simulink model "MotorTorqueControlTest_working_5_8_2022_ADC_FILT_Mo"  (R2024b)
settings: Solver=FixedStepAuto  StartTime=0.0  StopTime=inf  FixedStep=0.001  RelTol=1e-3  EnableMultiTasking=on
undefined symbols (not defined in the file): mu_X, mu_y, sigma_X, sigma_y
libraries: slrealtimeethercatlib x35, slrealtimeiplib x6, slrealtimeutilitieslib x5, simulink_extras x5, slrealtimeloglib x3, slpidlib x1, simulink x1
(part 1 of 4)
settings Model: SimulationMode=external  ExtModeEnableFloating=off  Creator=mbout  LastModifiedBy=Andy
settings SolverCC: ConcurrentTasks=on  AlgebraicLoopSolver=TrustRegion  PositivePriorityOrder=on  AutoInsertRateTranBlk=on  InsertRTBMode=Never (minimum delay)
settings DataIOCC: SaveFormat=Array  SaveState=on  SignalLoggingName=logsOut
settings OptimizationCC: BlockReduction=off  BooleanDataType=off  OptimizeBlockIOStorage=off  BufferReuse=off  ReuseModelBlockBuffer=off  GlobalBufferReuse=off  ExpressionFolding=off  LocalBlockOutputs=off  InitFltsAndDblsToZero=on  OptimizeDataStoreBuffers=off  BusAssignmentInplaceUpdate=off
settings DebuggingCC: SaveWithParameterizedLinksMsg=none  UnderspecifiedInitializationDetection=Classic  MergeDetectMultiDrivingBlocksExec=none  CheckExecutionContextPreStartOutputMsg=on  SignalResolutionControl=TryResolveAllWithWarning  TasksWithSamePriorityMsg=none  ParameterPrecisionLossMsg=none  UnconnectedInputMsg=warning  UnconnectedOutputMsg=warning  UnconnectedLineMsg=warning  SFUnexpectedBacktrackingDiag=warning  SFNoUnconditionalDefaultTransitionDiag=warning  SFExecutionAtInitializationDiag=none  UnderSpecifiedDimensionMsg=warning  ArithmeticOperatorsInVariantConditions=warning
settings HardwareCC: ProdBitPerLong=64  ProdLongLongMode=on  ProdHWDeviceType=Intel->x86-64 (Linux 64)
settings ModelReferenceCC: EnableRefExpFcnMdlSchedulingChecks=on  PropagateSignalLabelsOutOfModel=off
settings SFSimCC: SimUseLocalCustomCode=off  SimTargetLang=C++
settings RTWCC: Description=Speedgoat Real-Time Target Machine  SystemTargetFile=speedgoat.tlc  TemplateMakefile=slrealtime_default_tmf  RTWUseLocalCustomCode=off  Toolchain=Simulink Real-Time Toolchain  BuildConfiguration=Faster Runs  CodeExecutionProfiling=on  TargetLang=C++  GPUComputeCapability=3.5  DLArmComputeVersion=19.05
settings CodeAppCC: StateflowObjectComments=on
settings SimulinkRealTimeTargetCC: InstructionSetFMA=off  LogToMDFFile=off  SLRTFileLogMaxRuns=20
settings ConfigComp: CovMetricSettings=dw  CovSaveCumulativeToWorkspaceVar=on  CovSaveSingleToWorkspaceVar=on  CovExternalEMLEnable=off  CovSFcnEnable=off

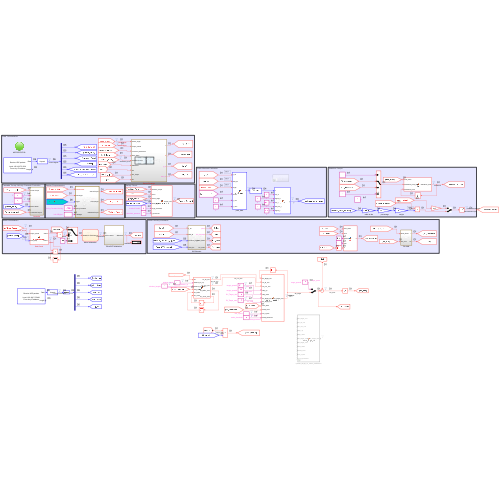
[thumbnail: Simulink's stored preview of the top-level diagram]
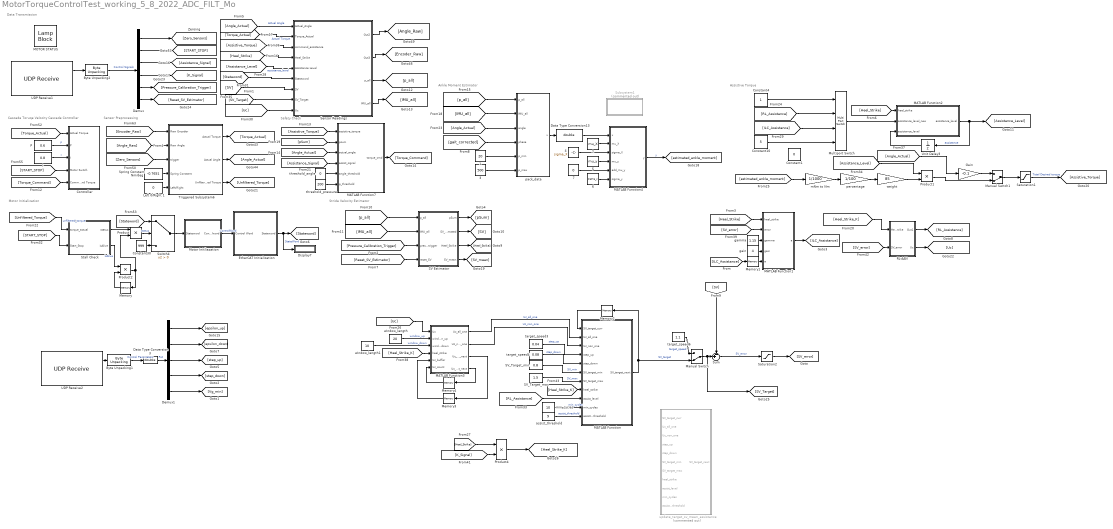
== system MotorTorqueControlTest_working_5_8_2022_ADC_FILT_Mo ==
  note: Ankle Moment Estimator
  note: Cascade Toruqe Velocity Cascade Controller
  note: Data Transmission
  note: Motor Initialization
  note: Sensor Preprocessing
  note: Stride Velocity Estimator
  note: Assistive Torque
  note: Safety Check
  1 : Constant  Value=20
  2 : Constant  Value=mu_X
  3 : Constant  Value=500
  4 : Constant  Value=sigma_X
  5 : Constant  Value=mu_y
  6 : Constant  Value=sigma_y
  7 : Constant  Value=0
  Byte Unpacking1 : slrealtimeutilitieslib/Byte Unpacking  MaskUnpackedDataTypes={['single']}  MaskUnpackedDataSizes={[6]}  MaskAlignment=1
  Byte Unpacking2 : slrealtimeutilitieslib/Byte Unpacking  MaskUnpackedDataTypes={['single']}  MaskUnpackedDataSizes={[6]}  MaskAlignment=1
  Constant1 : Constant  Value=0
  Constant10 : Constant  Value=5
  Constant30 : Constant  Value=999
  Constant4 : Constant
  Controller : Subsystem
  Data Type Conversion13 : DataTypeConversion  OutDataTypeStr=double  SaturateOnIntegerOverflow=off  RndMeth=Floor
  Data Type Conversion3 : DataTypeConversion  OutDataTypeStr=double  SaturateOnIntegerOverflow=off  RndMeth=Floor
  Demux : Demux  Outputs=6
  Demux1 : Demux  Outputs=5
  Display7 : Display
  EtherCAT Initialization : Subsystem
  Gain : Gain  Gain=-0.1
  I : Constant  Value=0.8
  Left 0/Right 1 : Constant  Value=0
  MATLAB Function : MATLAB Function  TreatAsAtomicUnit=on
  MATLAB Function1 : MATLAB Function  TreatAsAtomicUnit=on
  MATLAB Function2 : MATLAB Function  TreatAsAtomicUnit=on
  MATLAB Function3 : MATLAB Function  TreatAsAtomicUnit=on
  MATLAB Function4 : MATLAB Function  TreatAsAtomicUnit=on  SystemSampleTime=0.01
  MATLAB Function7 : MATLAB Function  TreatAsAtomicUnit=on  SystemSampleTime=0.001
  MOTOR STATUS : LampBlock  LabelPosition=Hide
  Manual Switch : ManualSwitch  CurrentSetting=0
  Manual Switch1 : ManualSwitch  CurrentSetting=0
  Memory : Memory  InitialCondition=1
  Memory1 : Memory
  Memory2 : Memory  InitialCondition=0.5
  Memory3 : Memory  InitialCondition=zeros(60,1)
  Memory4 : Memory  InitialCondition=zeros(2,1)
  Motor Initliazation : Stateflow chart  TreatAsAtomicUnit=on
  Multiport Switch : MultiPortSwitch  SaturateOnIntegerOverflow=off  InputSameDT=off
  P : Constant  Value=0.6
  Product{,1..2,4} (4 alike) : Product
  RL-AAN : Subsystem
  SV Estimator : Subsystem
  SV_Target_max : Constant  Value=1.5
  SV_Target_min : Constant  Value=0.8
  Saturation1 : Saturate  UpperLimit=8  LowerLimit=0
  Saturation2 : Saturate  UpperLimit=inf  LowerLimit=0
  Sensor Readings : Subsystem
  Spring Constant Nm/deg : Constant  Value=-0.7651
  Stall Check : MATLAB Function  TreatAsAtomicUnit=on
  Subsystem1 : Subsystem  Commented=on
  Sum : Sum  Inputs=-+|
  Switch4 : Switch  Criteria=u2 > Threshold  SaturateOnIntegerOverflow=off  InputSameDT=off
  Triggered Subsystem6 : Subsystem  TreatAsAtomicUnit=on
  UDP Receive1 : slrealtimeiplib/UDP Receive  useHostTargetConn=off  ipAddress=192.168.7.5  localPort=5431  rcvWidth=24  rcvFmAny=on  fmAddress='10.10.10.10'  sampleTime=0.1  enableMessage=off  maxPackets=1
  UDP Receive2 : slrealtimeiplib/UDP Receive  useHostTargetConn=off  ipAddress=192.168.7.5  localPort=5430  rcvWidth=24  rcvFmAny=on  fmAddress='10.10.10.10'  sampleTime=0.1  enableMessage=off  maxPackets=1
  Unit Delay3 : UnitDelay  SampleTime=-1
  assist_threshold : Constant  Value=9
  gain : Constant  Value=4
  gamma : Constant  Value=1.15
  mNm to Nm : Gain  Gain=1/1000
  min_cycles : Constant  Value=10
  pack_data : MATLAB Function  TreatAsAtomicUnit=on  SystemSampleTime=0.01
  percentage : Gain  Gain=1/100
  target_speed3 : Constant  Value=0.04
  target_speed4 : Constant  Value=0.08
  target_speed6 : Constant  Value=1.1
  threshold_angle : Constant  Value=0
  threshold_pressure : Constant  Value=200
  update_target_sv_mean_assistance : MATLAB Function  Commented=on  TreatAsAtomicUnit=on
  weight : Gain  Gain=85
  window_length : Constant  Value=20
  window_length1 : Constant  Value=10
  wires:
  EtherCAT Initialization/1(Stateword) -> [Stateword], Display7/1  "StateWord"
  [Zero_Sensors] -> Triggered Subsystem6/3(trigger)
  Sensor Readings/2(Out3) -> [Encoder_Raw]
  Triggered Subsystem6/2(Actual Angle) -> [Angle_Actual]
  Motor Initliazation/1(Controlword) -> EtherCAT Initialization/1(Control Word)  "ControlWord"
  [Encoder_Raw] -> Triggered Subsystem6/1(Raw Encoder)
  [Torque_Actual] -> Controller/1(Actual Torque)
  [START_STOP] -> Controller/4(Motor Switch)
  [Angle_Raw] -> Triggered Subsystem6/2(Raw Angle)
  Sensor Readings/1(Out2) -> [Angle_Raw]
  [Stateword] -> Switch4/1
  Constant30/1 -> Switch4/3
  P/1 -> Controller/2(P)  "P"
  I/1 -> Controller/3(I)  "I"
  MATLAB Function7/1(torque_cmd) -> [Torque_Command]
  Triggered Subsystem6/1(Actual Torque) -> [Torque_Actual]
  Saturation1/1 -> [Assistive_Torque]  "Total Desired torque"
  gain/1 -> MATLAB Function1/4(gain)
  gamma/1 -> MATLAB Function1/3(gamma)
  [SV] -> Sum/1
  Memory1/1 -> MATLAB Function1/5("a ")
  MATLAB Function1/1(a) -> [ILC_Assistance]
  [Angle_Actual] -> Sensor Readings/1(Actual_Angle)  "Actual Angle"
  [Torque_Actual] -> Sensor Readings/2(Torque_Actual)  "Actual Torque"
  percentage/1 -> weight/1
  [Assistive_Torque] -> Sensor Readings/3(command_assistance)
  mNm to Nm/1 -> percentage/1
  weight/1 -> Product1/2
  [RL_Assistance] -> Multiport Switch/2
  MATLAB Function4/1(y) -> [estimated_ankle_moment]  "y"
  Sensor Readings/3(p_all) -> [p_all]
  Sensor Readings/4(IMU_all) -> [IMU_all]
  [p_all] -> pack_data/1(p_all)
  [Angle_Actual] -> pack_data/3(angle)
  [gait_corrected] -> pack_data/4(phase)
  1/1 -> pack_data/5(p_min)
  3/1 -> pack_data/6(p_max)
  [estimated_ankle_moment] -> mNm to Nm/1
  MATLAB Function2/1(assistance_level) -> [Assistance_Level], Unit Delay3/1  "assistance"
  Unit Delay3/1 -> MATLAB Function2/3("assistance_level ")
  [Assistance_Level] -> Sensor Readings/5(Assistance Level)  "assistance_level"
  Constant10/1 -> Multiport Switch/4
  2/1 -> MATLAB Function4/2(mu_X)
  4/1 -> MATLAB Function4/3(sigma_X)
  5/1 -> MATLAB Function4/4(mu_y)
  6/1 -> MATLAB Function4/6(sigma_y)
  7/1 -> MATLAB Function4/5(add_mu_y)
  pack_data/1(x) -> Data Type Conversion13/1
  Data Type Conversion13/1 -> MATLAB Function4/1(x)
  [ILC_Assistance] -> Multiport Switch/3
  [Heel_Strike] -> MATLAB Function1/1(heel_strike)
  [IMU_all] -> pack_data/2(IMU_all)
  [START_STOP] -> Stall Check/2(Start_Stop)
  [Unfiltered_Torque] -> Stall Check/1(torque_actual)  "unfiltered_torque"
  Byte Unpacking2/1 -> Demux/1  "Control Signals"
  Demux/1 -> [Zero_Sensors]
  Demux/2 -> [START_STOP]
  Demux/3 -> [Assistance_Signal]
  Demux/4 -> [K_Signal]
  [Stateword] -> Sensor Readings/6(Stateword)
  UDP Receive1/1 -> Byte Unpacking2/1
  Demux/6 -> [Reset_SV_Estimator]
  Demux/5 -> [Pressure_Calibration_Trigger]
  [Heel_Strike] -> Sensor Readings/4(Heel_Strike)
  [Assistance_Level] -> Product1/1
  Constant4/1 -> Multiport Switch/1
  Multiport Switch/1 -> MATLAB Function2/2(assistance_level_new)
  [Heel_Strike] -> MATLAB Function2/1(heel_strike)
  [SV_error] -> MATLAB Function1/2(error)
  Saturation2/1 -> [SV_error]
  Sum/1 -> Saturation2/1  "SV_error"
  SV_Target_max/1 -> MATLAB Function/7(SV_target_max)  "SV_max"
  [SV_error] -> RL-AAN/2(SV_error)
  RL-AAN/1(Out1) -> [RL_Assistance]
  [Pressure_Calibration_Trigger] -> SV Estimator/3(pressure_trigger)
  [Reset_SV_Estimator] -> SV Estimator/4(reset_SV)
  SV Estimator/1(pSum) -> [pSum]
  SV Estimator/3(Heel_Strike) -> [Heel_Strike]
  SV Estimator/2(SV_estimated) -> [SV]
  [p_all] -> SV Estimator/1(p_all)
  [IMU_all] -> SV Estimator/2(IMU_all)
  [Torque_Command] -> Controller/5(Command Torque)
  Spring Constant Nm/deg/1 -> Triggered Subsystem6/4(Spring Constant)
  Switch4/1 -> Motor Initliazation/1(Stateword)
  Stall Check/1(status) -> Product/1
  [pSum] -> MATLAB Function7/2(psum)
  [Angle_Actual] -> MATLAB Function7/3(actual_angle)
  [Assistance_Signal] -> MATLAB Function7/4(assist_signal)
  threshold_pressure/1 -> MATLAB Function7/6(p_threshold)
  threshold_angle/1 -> MATLAB Function7/5(angle_threshold)
  [Assistive_Torque] -> MATLAB Function7/1(assistive_torque)
  [ILC_Assistance] -> Memory1/1
  Left 0/Right 1/1 -> Triggered Subsystem6/5(Left/Right)
  MATLAB Function/1(SV_target_next) -> Manual Switch/2, Memory2/1  "SV_target"
  target_speed3/1 -> MATLAB Function/4(step_up)  "step_up"
  target_speed4/1 -> MATLAB Function/5(step_down)  "step_down"
  SV_Target_min/1 -> MATLAB Function/6(SV_target_min)  "SV_min"
  Demux1/2 -> [epsilon_down]
  Demux1/3 -> [step_up]
  Demux1/1 -> [epsilon_up]
  Demux1/4 -> [step_down]
  UDP Receive2/1 -> Byte Unpacking1/1
  Byte Unpacking1/1 -> Data Type Conversion3/1  "Control Parameters"
  Demux1/5 -> [Vg_min]
  Data Type Conversion3/1 -> Demux1/1  "Pot"
  [SV] -> Sensor Readings/7(SV)
  SV Estimator/4(SV_mean) -> [SV_mean]
  target_speed6/1 -> Manual Switch/1  "target_speed"
  Manual Switch/1 -> [SV_Target], Sum/2
  Triggered Subsystem6/3(Unfiltered Torque) -> [Unfiltered_Torque]
  Stall Check/2(isAlive) -> Product2/1  "isAlive"
  Memory/1 -> Product2/2
  Product2/1 -> Memory/1, Product/2
  Product/1 -> Switch4/2  "status"
  RL-AAN/2(Uc) -> [Uc]
  [Uc] -> MATLAB Function3/1(Uc)
  MATLAB Function3/3(Uc_buffer_next) -> Memory3/1
  Memory3/1 -> MATLAB Function3/5(Uc_buffer)
  window_length/1 -> MATLAB Function3/2(window_len_up)  "window_up"
  MATLAB Function3/2(Uc_non_one) -> MATLAB Function/3(Uc_non_one)  "Uc_non_one"
  MATLAB Function3/1(Uc_all_one) -> MATLAB Function/2(Uc_all_one)  "Uc_all_one"
  Memory2/1 -> MATLAB Function/1(SV_target_curr)
  MATLAB Function3/4(Uc_count_next) -> Memory4/1
  Memory4/1 -> MATLAB Function3/6(Uc_count)
  window_length1/1 -> MATLAB Function3/3(window_len_down)  "window_down"
  [SV_Target] -> Sensor Readings/8(SV_Target)
  [Uc] -> Sensor Readings/9(Uc)
  [K_Signal] -> Product4/2
  Product4/1 -> [Heel_Strike_K]
  [Heel_Strike] -> Product4/1
  [Heel_Strike_K] -> MATLAB Function3/4(heel_strike)
  [Heel_Strike_K] -> MATLAB Function/8(heel_strike)
  [Heel_Strike_K] -> RL-AAN/1(Heel_Strike)
  Product1/1 -> Manual Switch1/2
  min_cycles/1 -> MATLAB Function/10(min_cycles)  "min_cycles"
  assist_threshold/1 -> MATLAB Function/11(assist_threshold)  "assist_threshold"
  [RL_Assistance] -> MATLAB Function/9(assist_level)
  Manual Switch1/1 -> Saturation1/1
  Gain/1 -> Manual Switch1/1
  [Angle_Actual] -> Gain/1

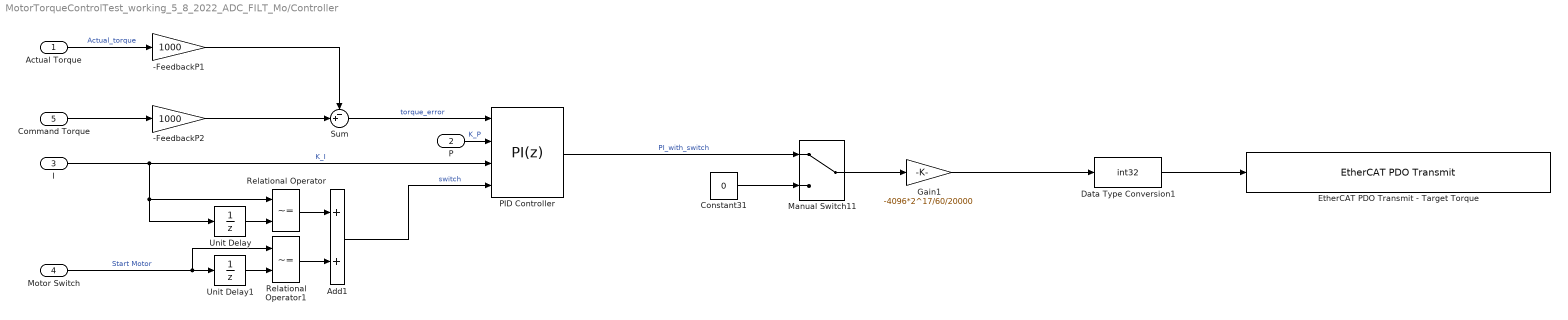
== system MotorTorqueControlTest_working_5_8_2022_ADC_FILT_Mo/Controller ==
  Actual Torque : Inport
  P : Inport  Port=2
  I : Inport  Port=3
  Motor Switch : Inport  Port=4
  Command Torque : Inport  Port=5
  -FeedbackP1 : Gain  Gain=1000
  -FeedbackP2 : Gain  Gain=1000
  Add1 : Sum
  Constant31 : Constant  Value=0
  Data Type Conversion1 : DataTypeConversion  OutDataTypeStr=int32  SaturateOnIntegerOverflow=off  RndMeth=Floor
  EtherCAT PDO Transmit - Target Torque : slrealtimeethercatlib/EtherCAT PDO Transmit  Priority=3  sig_name=Drive 1 (AMC Servo Drive).Outputs.Target Velocity  sig_offset=328  sig_type=int32  type_size=32  sig_dim=1  device_id=0  sample_time=0.001000
  Gain1 : Gain  Gain=-4096*2^17/60/20000
  Manual Switch11 : ManualSwitch
  PID Controller : slpidlib/PID Controller  Controller=PI  Form=Parallel  TimeDomain=Discrete-time  UseExternalTs=off  SampleTime=-1  IntegratorMethod=Forward Euler  FilterMethod=Forward Euler  ControllerParametersSource=external  P=1  I=1  UseKiTs=off  D=0  UseExternalDerivativeSource=off  N=100  UseFilter=on  TunerSelectOption=Transfer Function Based (PID Tuner App)  InitialConditionSource=internal  InitialConditionForIntegrator=0  InitialConditionForFilter=0  DifferentiatorICPrevScaledInput=0  ExternalReset=either  TrackingMode=off  Kt=1  LimitOutput=off  SatLimitsSource=internal  UpperSaturationLimit=50  LowerSaturationLimit=-50  LinearizeAsGain=on  AntiWindupMode=none  Kb=1  LimitIntegrator=off  UpperIntegratorSaturationLimit=inf  LowerIntegratorSaturationLimit=-inf  POutMin=[]  POutMax=[]  IOutMin=[]  IOutMax=[]  DOutMin=[]  DOutMax=[]  NOutMin=[]  NOutMax=[]  SumOutMin=[]  SumOutMax=[]  SaturationOutMin=[]  SaturationOutMax=[]  PParamMin=[]  PParamMax=[]  IParamMin=[]  IParamMax=[]  DParamMin=[]  DParamMax=[]  NParamMin=[]  NParamMax=[]  KbParamMin=[]  KbParamMax=[]  KtParamMin=[]  KtParamMax=[]  KbOutMin=[]  KbOutMax=[]  KtOutMin=[]  KtOutMax=[]  IntegratorOutMin=[]  IntegratorOutMax=[]  FilterOutMin=[]  FilterOutMax=[]  SumI1OutMin=[]  SumI1OutMax=[]  SumI2OutMin=[]  SumI2OutMax=[]  SumI3OutMin=[]  SumI3OutMax=[]  SumI4OutMin=[]  SumI4OutMax=[]  SumDOutMin=[]  SumDOutMax=[]  DifferentiatorOutMin=[]  DifferentiatorOutMax=[]  FilterDiffOutCoefMin=[]  FilterDiffOutCoefMax=[]  ReciprocalOutMin=[]  ReciprocalOutMax=[]  SumDenOutMin=[]  SumDenOutMax=[]  SumNumOutMin=[]  SumNumOutMax=[]  DivideOutMin=[]  DivideOutMax=[]  UdiffTsProdOutMin=[]  UdiffTsProdOutMax=[]  NTsProdOutMin=[]  NTsProdOutMax=[]  UintegralTsProdOutMin=[]  UintegralTsProdOutMax=[]  UngainTsProdOutMin=[]  UngainTsProdOutMax=[]  ClampingZeroOutDataTypeStr=Inherit: Inherit via back propagation  ClampingZeroOutMin=[]  ClampingZeroOutMax=[]  FilterDenConstantOutDataTypeStr=Inherit: Inherit via back propagation  FilterDenConstantOutMin=[]  FilterDenConstantOutMax=[]  PCopyOutDataTypeStr=Inherit: Inherit via back propagation  PCopyOutMin=[]  PCopyOutMax=[]  NCopyOutDataTypeStr=Inherit: Inherit via back propagation  NCopyOutMin=[]  NCopyOutMax=[]  IntegratorContinuousStateAttributes=''  IntegratorStateMustResolveToSignalObject=off  IntegratorRTWStateStorageClass=Auto  FilterContinuousStateAttributes=''  FilterStateMustResolveToSignalObject=off  FilterRTWStateStorageClass=Auto  ParallelPVariant=ExternalParameters  IdealPVariant=Disabled  IVariant=ExternalParameters  DVariant=Disabled  IntegratorVariant=Discrete  SatVariant=Disabled  AWVariant=Passthrough  PCopyVariant=Disabled  TRVariant=Disabled  FdbkBlocksVariant=Forward  IdealPFdbkVariant=Disabled  SatFdbkVariant=Disabled  DerivativeFilterVariant=Disabled  NVariant=Disabled  NCopyVariant=Disabled_SignalSpec  FilterICVariant=Disabled  IntegratorICVariant=InternalICs  ExternalResetVariant=ExternalReset  TRSumVariant=Passthrough  SumFdbkVariant=Disabled  SumVariant=Sum_PI  TsampFilterVariant=InternalTs  TsampNgainVariant=Passthrough  TsampIntegralVariant=Disabled_SignalSpec  ExternalSaturationOutDataTypeStr=Inherit: Same as second input  DerivativeSourceVariant=Disabled  PreIntVariant=InternalPreInt
  Relational Operator : RelationalOperator  Operator=~=  OutDataTypeStr=boolean  RndMeth=Simplest  InputSameDT=off
  Relational Operator1 : RelationalOperator  Operator=~=  OutDataTypeStr=boolean  RndMeth=Simplest  InputSameDT=off
  Sum : Sum  Inputs=-+|
  Unit Delay : UnitDelay  SampleTime=-1  HasFrameUpgradeWarning=on
  Unit Delay1 : UnitDelay  SampleTime=-1  HasFrameUpgradeWarning=on
  wires:
  Data Type Conversion1/1 -> EtherCAT PDO Transmit - Target Torque/1
  Motor Switch/1 -> Unit Delay1/1, Relational Operator1/1  "Start Motor"
  Unit Delay/1 -> Relational Operator/2
  Unit Delay1/1 -> Relational Operator1/2
  Relational Operator/1 -> Add1/1
  Relational Operator1/1 -> Add1/2
  Command Torque/1 -> -FeedbackP2/1
  -FeedbackP2/1 -> Sum/2
  -FeedbackP1/1 -> Sum/1
  Actual Torque/1 -> -FeedbackP1/1  "Actual_torque"
  I/1 -> Unit Delay/1, Relational Operator/1, PID Controller/3  "K_I"
  Sum/1 -> PID Controller/1  "torque_error"
  P/1 -> PID Controller/2  "K_P"
  Add1/1 -> PID Controller/4  "switch"
  PID Controller/1 -> Manual Switch11/1  "PI_with_switch"
  Constant31/1 -> Manual Switch11/2
  Manual Switch11/1 -> Gain1/1
  Gain1/1 -> Data Type Conversion1/1

== system MotorTorqueControlTest_working_5_8_2022_ADC_FILT_Mo/EtherCAT Initialization ==
  note: This block is used for the initialization of the EtherCAT network. The block points the model to the folder location of the ENI file created in TwinCAT. Note that the ENI file must also be present in the simulink's model directory, and the name of the ENI file must be different from the simulink model.
  note: This block and associated scope is used to show the state of the EtherCAT State Machine. Clicking "Help" in the Get State block shows the status numbers and their corresponding states. The scope can be helpful for determing the state and troubleshooting if the drive is not enabling and the motor is not turning on.
  note: This block and associated scope is used to show the status word of the drive's state machine. Note that the drive's state machine is different from the EtherCAT State Machine described above. This scope is also helpful for troubleshooting. Note that the status word is given as a decimal number and must be converted to binary to decipher its meaning.
  note: The control word is the PDO that changes the state of the motor. Refer to the EPOS library for more information.
  Control Word : Inport
  Constant2 : Constant  Value=9
  Data Type Conversion : DataTypeConversion  OutDataTypeStr=uint16  SaturateOnIntegerOverflow=off  RndMeth=Floor
  Data Type Conversion1 : DataTypeConversion  OutDataTypeStr=uint16  SaturateOnIntegerOverflow=off  RndMeth=Floor
  Display : Display
      settings: Format=hex (Stored Integer)
  Display1 : Display
  Display2 : Display
  EtherCAT Get State : slrealtimeethercatlib/EtherCAT Get State  device_id=0  sample_time=0
  EtherCAT Init : slrealtimeethercatlib/EtherCAT Init  Priority=0  config_file=C:\Users\Andy\Desktop\AFO\PDO__AMC_Drive_32_Input.xml  device_id=0  portnum=1  initstate=2  dctuning=2  enaDebug=1  logFile='c:\dbglog.txt'  sample_time=0.001000  DCMode=0
  EtherCAT PDO Receive : slrealtimeethercatlib/EtherCAT PDO Receive  Priority=2  sig_name=Drive 1 (AMC Servo Drive).Inputs.Status Word  sig_offset=312  sig_type=uint16  type_size=16  sig_dim=1  device_id=0  sample_time=0.001000
  EtherCAT PDO Transmit : slrealtimeethercatlib/EtherCAT PDO Transmit  Priority=3  sig_name=Drive 1 (AMC Servo Drive).Outputs.Control Word  sig_offset=312  sig_type=uint16  type_size=16  sig_dim=1  device_id=0  sample_time=0.001000
  EtherCAT PDO Transmit1 : slrealtimeethercatlib/EtherCAT PDO Transmit  Priority=3  sig_name=Drive 1 (AMC Servo Drive).Outputs.Modes of Operation  sig_offset=360  sig_type=uint16  type_size=16  sig_dim=1  device_id=0  sample_time=0.001000
  Stateword : Outport
  wires:
  EtherCAT PDO Receive/1 -> Stateword/1, Display2/1
  EtherCAT Get State/1 -> Display1/1
  EtherCAT Init/1 -> Display/1
  Data Type Conversion/1 -> EtherCAT PDO Transmit/1
  Control Word/1 -> Data Type Conversion/1
  Constant2/1 -> Data Type Conversion1/1
  Data Type Conversion1/1 -> EtherCAT PDO Transmit1/1

== system MotorTorqueControlTest_working_5_8_2022_ADC_FILT_Mo/RL-AAN ==
  Heel_Strike : Inport
  SV_error : Inport  Port=2
  Byte Unpacking1 : slrealtimeutilitieslib/Byte Unpacking  MaskUnpackedDataTypes={['double']}  MaskUnpackedDataSizes={[2]}  MaskAlignment=1
  Demux1 : Demux  Outputs=2
  RT : RateTransition  Deterministic=off  OutPortSampleTime=0.001
  Saturation : Saturate  UpperLimit=10  LowerLimit=0
  Triggered Subsystem : Subsystem  TreatAsAtomicUnit=on
  UDP RL_AAN : slrealtimeiplib/UDP Receive  useHostTargetConn=off  ipAddress=192.168.7.5  localPort=6009  rcvWidth=16  rcvFmAny=on  fmAddress='10.10.10.10'  sampleTime=0.1  enableMessage=off  maxPackets=1
  Out1 : Outport
  Uc : Outport  Port=2
  wires:
  SV_error/1 -> Triggered Subsystem/1(In1)
  Heel_Strike/1 -> Triggered Subsystem/Trigger
  Saturation/1 -> Out1/1  "RL_AAN"
  Byte Unpacking1/1 -> RT/1
  UDP RL_AAN/1 -> Byte Unpacking1/1
  Demux1/1 -> Saturation/1
  Demux1/2 -> Uc/1  "Uc"
  RT/1 -> Demux1/1

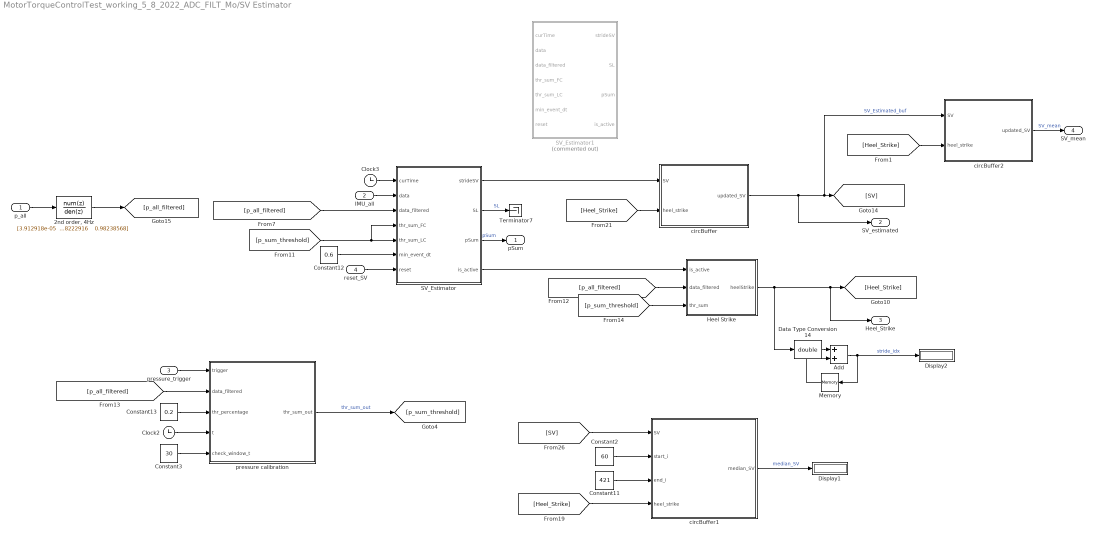
== system MotorTorqueControlTest_working_5_8_2022_ADC_FILT_Mo/SV Estimator ==
  p_all : Inport
  IMU_all : Inport  Port=2
  pressure_trigger : Inport  Port=3
  reset_SV : Inport  Port=4
  "2nd order, 4Hz" : DiscreteFilter  Numerator="[3.912918e-05  7.825836e-05   3.912918e-05]"  Denominator="[1.0000   -1.98222916    0.98238568]"
  Add : Sum
  Clock2 : Clock
  Clock3 : Clock
  Constant11 : Constant  Value=421
  Constant12 : Constant  Value=0.6
  Constant13 : Constant  Value=0.2
  Constant2 : Constant  Value=60
  Constant3 : Constant  Value=30
  Data Type Conversion14 : DataTypeConversion  OutDataTypeStr=double  SaturateOnIntegerOverflow=off  RndMeth=Floor
  Display1 : Display
  Display2 : Display
  Heel Strike : MATLAB Function  TreatAsAtomicUnit=on  SystemSampleTime=0.001
  Memory : Memory
  SV_Estimator : MATLAB Function  TreatAsAtomicUnit=on  SystemSampleTime=0.001
  SV_Estimator1 : MATLAB Function  Commented=on  TreatAsAtomicUnit=on  SystemSampleTime=0.001
  Terminator7 : Terminator
  circBuffer : MATLAB Function  TreatAsAtomicUnit=on  SystemSampleTime=0.001
  circBuffer1 : MATLAB Function  TreatAsAtomicUnit=on  SystemSampleTime=0.001
  circBuffer2 : MATLAB Function  TreatAsAtomicUnit=on  SystemSampleTime=0.001
  pressure calibration : MATLAB Function  TreatAsAtomicUnit=on  SystemSampleTime=0.001
  pSum : Outport
  SV_estimated : Outport  Port=2
  Heel_Strike : Outport  Port=3
  SV_mean : Outport  Port=4
  wires:
  "2nd order, 4Hz"/1 -> [p_all_filtered]
  [p_sum_threshold] -> Heel Strike/3(thr_sum)
  [p_sum_threshold] -> SV_Estimator/4(thr_sum_FC), SV_Estimator/5(thr_sum_LC)
  SV_Estimator/3(pSum) -> pSum/1  "pSum"
  pressure calibration/1(thr_sum_out) -> [p_sum_threshold]  "thr_sum_out"
  SV_Estimator/1(strideSV) -> circBuffer/1(SV)
  Clock2/1 -> pressure calibration/4(t)
  Constant2/1 -> circBuffer1/2(start_i)
  reset_SV/1 -> SV_Estimator/7(reset)
  circBuffer1/1(median_SV) -> Display1/1  "median_SV"
  SV_Estimator/4(is_active) -> Heel Strike/1(is_active)
  [Heel_Strike] -> circBuffer1/4(heel_strike)
  SV_Estimator/2(SL) -> Terminator7/1  "SL"
  circBuffer/1(updated_SV) -> circBuffer2/1(SV), [SV], SV_estimated/1  "SV_Estimated_buf"
  [p_all_filtered] -> SV_Estimator/3(data_filtered)
  [Heel_Strike] -> circBuffer/2(heel_strike)
  [p_all_filtered] -> pressure calibration/2(data_filtered)
  IMU_all/1 -> SV_Estimator/2(data)
  Clock3/1 -> SV_Estimator/1(curTime)
  [SV] -> circBuffer1/1(SV)
  [p_all_filtered] -> Heel Strike/2(data_filtered)
  Constant3/1 -> pressure calibration/5(check_window_t)
  Constant11/1 -> circBuffer1/3(end_i)
  p_all/1 -> "2nd order, 4Hz"/1
  Constant13/1 -> pressure calibration/3(thr_percentage)
  Heel Strike/1(heelStrike) -> Data Type Conversion14/1, Heel_Strike/1, [Heel_Strike]
  pressure_trigger/1 -> pressure calibration/1(trigger)
  Constant12/1 -> SV_Estimator/6(min_event_dt)
  circBuffer2/1(updated_SV) -> SV_mean/1  "SV_mean"
  [Heel_Strike] -> circBuffer2/2(heel_strike)
  Add/1 -> Memory/1, Display2/1  "stride_idx"
  Memory/1 -> Add/2
  Data Type Conversion14/1 -> Add/1

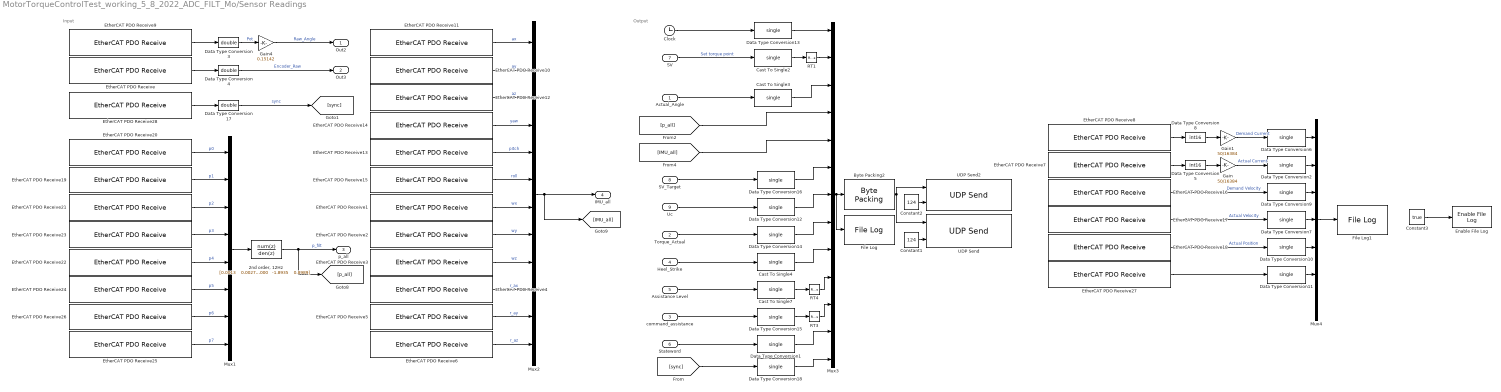
== system MotorTorqueControlTest_working_5_8_2022_ADC_FILT_Mo/Sensor Readings ==
  note: Input
  note: Output
  Actual_Angle : Inport
  Torque_Actual : Inport  Port=2
  command_assistance : Inport  Port=3
  Heel_Strike : Inport  Port=4
  Assistance Level : Inport  Port=5
  Stateword : Inport  Port=6
  SV : Inport  Port=7
  SV_Target : Inport  Port=8
  Uc : Inport  Port=9
  "2nd order, 12Hz" : DiscreteFilter  Numerator="[0.0013    0.0027    0.0013]"  Denominator="[1.0000   -1.8935    0.8989]"
  Byte Packing2 : slrealtimeutilitieslib/Byte Packing  MaskPackedDataType=uint8  MaskUnpackedDataTypes={['single']}  MaskAlignment=1
  Cast To Single{2..4,7} (4 alike) : DataTypeConversion  OutDataTypeStr=single  SaturateOnIntegerOverflow=off  RndMeth=Floor
  Clock : Clock
  Constant1 : Constant  Value=124
  Constant2 : Constant  Value=124
  Constant3 : Constant  Value=true
  Data Type Conversion{1..2,6..7,9..16,18} (13 alike) : DataTypeConversion  OutDataTypeStr=single  SaturateOnIntegerOverflow=off  RndMeth=Floor
  Data Type Conversion17 : DataTypeConversion  OutDataTypeStr=double  SaturateOnIntegerOverflow=off  RndMeth=Floor
  Data Type Conversion3 : DataTypeConversion  OutDataTypeStr=double  SaturateOnIntegerOverflow=off  RndMeth=Floor
  Data Type Conversion4 : DataTypeConversion  OutDataTypeStr=double  SaturateOnIntegerOverflow=off  RndMeth=Floor
  Data Type Conversion5 : DataTypeConversion  OutDataTypeStr=int16  SaturateOnIntegerOverflow=off  RndMeth=Floor
  Data Type Conversion8 : DataTypeConversion  OutDataTypeStr=int16  SaturateOnIntegerOverflow=off  RndMeth=Floor
  Enable File Log : slrealtimeloglib/Enable File Log
  EtherCAT PDO Receive : slrealtimeethercatlib/EtherCAT PDO Receive  Priority=2  sig_name=Box 2 (teensySensoryMB).Inputs.Force2  sig_offset=616  sig_type=single  type_size=32  sig_dim=1  device_id=0  sample_time=0.001000
  EtherCAT PDO Receive1 : slrealtimeethercatlib/EtherCAT PDO Receive  Priority=2  sig_name=Box 2 (teensySensoryMB).Inputs.Force24  sig_offset=1320  sig_type=single  type_size=32  sig_dim=1  device_id=0  sample_time=0.001000
  EtherCAT PDO Receive10 : slrealtimeethercatlib/EtherCAT PDO Receive  Priority=2  sig_name=Box 2 (teensySensoryMB).Inputs.Force22  sig_offset=1256  sig_type=single  type_size=32  sig_dim=1  device_id=0  sample_time=0.001000
  EtherCAT PDO Receive11 : slrealtimeethercatlib/EtherCAT PDO Receive  Priority=2  sig_name=Box 2 (teensySensoryMB).Inputs.Force21  sig_offset=1224  sig_type=single  type_size=32  sig_dim=1  device_id=0  sample_time=0.001000
  EtherCAT PDO Receive12 : slrealtimeethercatlib/EtherCAT PDO Receive  Priority=2  sig_name=Box 2 (teensySensoryMB).Inputs.Force23  sig_offset=1288  sig_type=single  type_size=32  sig_dim=1  device_id=0  sample_time=0.001000
  EtherCAT PDO Receive13 : slrealtimeethercatlib/EtherCAT PDO Receive  Priority=2  sig_name=Box 2 (teensySensoryMB).Inputs.Force10  sig_offset=872  sig_type=single  type_size=32  sig_dim=1  device_id=0  sample_time=0.001000
  EtherCAT PDO Receive14 : slrealtimeethercatlib/EtherCAT PDO Receive  Priority=2  sig_name=Box 2 (teensySensoryMB).Inputs.Force9  sig_offset=840  sig_type=single  type_size=32  sig_dim=1  device_id=0  sample_time=0.001000
  EtherCAT PDO Receive15 : slrealtimeethercatlib/EtherCAT PDO Receive  Priority=2  sig_name=Box 2 (teensySensoryMB).Inputs.Force11  sig_offset=904  sig_type=single  type_size=32  sig_dim=1  device_id=0  sample_time=0.001000
  EtherCAT PDO Receive16 : slrealtimeethercatlib/EtherCAT PDO Receive  Priority=2  sig_name=Drive 1 (AMC Servo Drive).Inputs.Velocity Demand  sig_offset=408  sig_type=int32  type_size=32  sig_dim=1  device_id=0  sample_time=0.001000
  EtherCAT PDO Receive17 : slrealtimeethercatlib/EtherCAT PDO Receive  Priority=2  sig_name=Drive 1 (AMC Servo Drive).Inputs.Actual Velocity  sig_offset=360  sig_type=int32  type_size=32  sig_dim=1  device_id=0  sample_time=0.001000
  EtherCAT PDO Receive18 : slrealtimeethercatlib/EtherCAT PDO Receive  Priority=2  sig_name=Drive 1 (AMC Servo Drive).Inputs.Actual Position  sig_offset=328  sig_type=int32  type_size=32  sig_dim=1  device_id=0  sample_time=0.001000
  EtherCAT PDO Receive19 : slrealtimeethercatlib/EtherCAT PDO Receive  Priority=2  sig_name=Box 2 (teensySensoryMB).Inputs.Force13  sig_offset=968  sig_type=single  type_size=32  sig_dim=1  device_id=0  sample_time=0.001000
  EtherCAT PDO Receive2 : slrealtimeethercatlib/EtherCAT PDO Receive  Priority=2  sig_name=Box 2 (teensySensoryMB).Inputs.Force25  sig_offset=1352  sig_type=single  type_size=32  sig_dim=1  device_id=0  sample_time=0.001000
  EtherCAT PDO Receive20 : slrealtimeethercatlib/EtherCAT PDO Receive  Priority=2  sig_name=Box 2 (teensySensoryMB).Inputs.Force12  sig_offset=936  sig_type=single  type_size=32  sig_dim=1  device_id=0  sample_time=0.001000
  EtherCAT PDO Receive21 : slrealtimeethercatlib/EtherCAT PDO Receive  Priority=2  sig_name=Box 2 (teensySensoryMB).Inputs.Force14  sig_offset=1000  sig_type=single  type_size=32  sig_dim=1  device_id=0  sample_time=0.001000
  EtherCAT PDO Receive22 : slrealtimeethercatlib/EtherCAT PDO Receive  Priority=2  sig_name=Box 2 (teensySensoryMB).Inputs.Force16  sig_offset=1064  sig_type=single  type_size=32  sig_dim=1  device_id=0  sample_time=0.001000
  EtherCAT PDO Receive23 : slrealtimeethercatlib/EtherCAT PDO Receive  Priority=2  sig_name=Box 2 (teensySensoryMB).Inputs.Force15  sig_offset=1032  sig_type=single  type_size=32  sig_dim=1  device_id=0  sample_time=0.001000
  EtherCAT PDO Receive24 : slrealtimeethercatlib/EtherCAT PDO Receive  Priority=2  sig_name=Box 2 (teensySensoryMB).Inputs.Force17  sig_offset=1096  sig_type=single  type_size=32  sig_dim=1  device_id=0  sample_time=0.001000
  EtherCAT PDO Receive25 : slrealtimeethercatlib/EtherCAT PDO Receive  Priority=2  sig_name=Box 2 (teensySensoryMB).Inputs.Force19  sig_offset=1160  sig_type=single  type_size=32  sig_dim=1  device_id=0  sample_time=0.001000
  EtherCAT PDO Receive26 : slrealtimeethercatlib/EtherCAT PDO Receive  Priority=2  sig_name=Box 2 (teensySensoryMB).Inputs.Force18  sig_offset=1128  sig_type=single  type_size=32  sig_dim=1  device_id=0  sample_time=0.001000
  EtherCAT PDO Receive27 : slrealtimeethercatlib/EtherCAT PDO Receive  Priority=2  sig_name=Drive 1 (AMC Servo Drive).Inputs.Status Word  sig_offset=312  sig_type=uint16  type_size=16  sig_dim=1  device_id=0  sample_time=0.001000
  EtherCAT PDO Receive28 : slrealtimeethercatlib/EtherCAT PDO Receive  Priority=2  sig_name=Box 2 (teensySensoryMB).Inputs.Force30  sig_offset=1512  sig_type=single  type_size=32  sig_dim=1  device_id=0  sample_time=0.001000
  EtherCAT PDO Receive3 : slrealtimeethercatlib/EtherCAT PDO Receive  Priority=2  sig_name=Box 2 (teensySensoryMB).Inputs.Force26  sig_offset=1384  sig_type=single  type_size=32  sig_dim=1  device_id=0  sample_time=0.001000
  EtherCAT PDO Receive4 : slrealtimeethercatlib/EtherCAT PDO Receive  Priority=2  sig_name=Box 2 (teensySensoryMB).Inputs.Force27  sig_offset=1416  sig_type=single  type_size=32  sig_dim=1  device_id=0  sample_time=0.001000
  EtherCAT PDO Receive5 : slrealtimeethercatlib/EtherCAT PDO Receive  Priority=2  sig_name=Box 2 (teensySensoryMB).Inputs.Force28  sig_offset=1448  sig_type=single  type_size=32  sig_dim=1  device_id=0  sample_time=0.001000
  EtherCAT PDO Receive6 : slrealtimeethercatlib/EtherCAT PDO Receive  Priority=2  sig_name=Box 2 (teensySensoryMB).Inputs.Force29  sig_offset=1480  sig_type=single  type_size=32  sig_dim=1  device_id=0  sample_time=0.001000
  EtherCAT PDO Receive7 : slrealtimeethercatlib/EtherCAT PDO Receive  Priority=2  sig_name=Drive 1 (AMC Servo Drive).Inputs.Actual Current  sig_offset=392  sig_type=int16  type_size=16  sig_dim=1  device_id=0  sample_time=0.001000
  EtherCAT PDO Receive8 : slrealtimeethercatlib/EtherCAT PDO Receive  Priority=2  sig_name=Drive 1 (AMC Servo Drive).Inputs.Iq - Demand  sig_offset=472  sig_type=uint16  type_size=16  sig_dim=1  device_id=0  sample_time=0.001000
  EtherCAT PDO Receive9 : slrealtimeethercatlib/EtherCAT PDO Receive  Priority=2  sig_name=Box 2 (teensySensoryMB).Inputs.Force4  sig_offset=680  sig_type=single  type_size=32  sig_dim=1  device_id=0  sample_time=0.001000
  File Log : slrealtimeloglib/File Log  decimation=1  inputProcessing=Elements as channels (sample based)
  File Log1 : slrealtimeloglib/File Log  decimation=1  inputProcessing=Elements as channels (sample based)
  Gain : Gain  Gain=50/16384
  Gain1 : Gain  Gain=50/16384
  Gain4 : Gain  Gain=0.15142
  Mux1 : Mux  Inputs=8
  Mux2 : Mux  Inputs=12
  Mux3 : Mux  Inputs=13
  Mux4 : Mux  Inputs=7
  RT1 : RateTransition  Deterministic=off  OutPortSampleTime=0.001
  RT3 : RateTransition  Deterministic=off  OutPortSampleTime=0.001
  RT4 : RateTransition  Deterministic=off  OutPortSampleTime=0.001
  UDP Send : slrealtimeiplib/UDP Send  useHostTargetConn=off  toAddress=192.168.7.15  toPort=5431  sampleTime=-1  enableMessage=off
  UDP Send2 : slrealtimeiplib/UDP Send  useHostTargetConn=off  toAddress='192.168.7.15'  toPort=5432  sampleTime=0.003  enableMessage=off
  Out2 : Outport
  Out3 : Outport  Port=2
  p_all : Outport  Port=3
  IMU_all : Outport  Port=4
  wires:
  Gain4/1 -> Out2/1  "Raw_Angle"
  EtherCAT PDO Receive9/1 -> Data Type Conversion3/1
  Data Type Conversion3/1 -> Gain4/1  "Pot"
  EtherCAT PDO Receive/1 -> Data Type Conversion4/1
  Data Type Conversion4/1 -> Out3/1  "Encoder_Raw"
  RT1/1 -> Mux3/2
  EtherCAT PDO Receive25/1 -> Mux1/8  "p7"
  EtherCAT PDO Receive12/1 -> Mux2/3  "az"
  EtherCAT PDO Receive15/1 -> Mux2/6  "roll"
  EtherCAT PDO Receive13/1 -> Mux2/5  "pitch"
  EtherCAT PDO Receive14/1 -> Mux2/4  "yaw"
  EtherCAT PDO Receive11/1 -> Mux2/1  "ax"
  EtherCAT PDO Receive10/1 -> Mux2/2  "ay"
  Actual_Angle/1 -> Cast To Single3/1
  Data Type Conversion14/1 -> Mux3/8
  command_assistance/1 -> Data Type Conversion15/1
  Torque_Actual/1 -> Data Type Conversion14/1
  Clock/1 -> Data Type Conversion13/1
  Data Type Conversion13/1 -> Mux3/1
  EtherCAT PDO Receive1/1 -> Mux2/7  "wx"
  EtherCAT PDO Receive2/1 -> Mux2/8  "wy"
  EtherCAT PDO Receive3/1 -> Mux2/9  "wz"
  EtherCAT PDO Receive4/1 -> Mux2/10  "r_ax"
  EtherCAT PDO Receive5/1 -> Mux2/11  "r_ay"
  EtherCAT PDO Receive6/1 -> Mux2/12  "r_az"
  Mux2/1 -> IMU_all/1, [IMU_all]
  Mux1/1 -> "2nd order, 12Hz"/1
  Cast To Single2/1 -> RT1/1
  Data Type Conversion15/1 -> RT3/1
  RT3/1 -> Mux3/11
  Cast To Single4/1 -> Mux3/9
  Assistance Level/1 -> Cast To Single7/1
  Cast To Single7/1 -> RT4/1
  RT4/1 -> Mux3/10
  Byte Packing2/1 -> UDP Send2/1, UDP Send/1
  Constant2/1 -> UDP Send2/2
  [p_all] -> Mux3/4
  Cast To Single3/1 -> Mux3/3
  [IMU_all] -> Mux3/5
  Constant1/1 -> UDP Send/2
  Data Type Conversion1/1 -> Mux3/12
  Heel_Strike/1 -> Cast To Single4/1
  SV/1 -> Cast To Single2/1  "Set torque point"
  Mux3/1 -> File Log/1, Byte Packing2/1
  EtherCAT PDO Receive20/1 -> Mux1/1  "p0"
  EtherCAT PDO Receive19/1 -> Mux1/2  "p1"
  EtherCAT PDO Receive21/1 -> Mux1/3  "p2"
  EtherCAT PDO Receive23/1 -> Mux1/4  "p3"
  EtherCAT PDO Receive22/1 -> Mux1/5  "p4"
  EtherCAT PDO Receive24/1 -> Mux1/6  "p5"
  EtherCAT PDO Receive26/1 -> Mux1/7  "p6"
  "2nd order, 12Hz"/1 -> [p_all], p_all/1  "p_filt"
  Constant3/1 -> Enable File Log/1
  Data Type Conversion6/1 -> Mux4/1
  Data Type Conversion2/1 -> Mux4/2
  Data Type Conversion9/1 -> Mux4/3
  Data Type Conversion7/1 -> Mux4/4
  EtherCAT PDO Receive16/1 -> Data Type Conversion9/1  "Demand Velocity"
  EtherCAT PDO Receive17/1 -> Data Type Conversion7/1  "Actual Velocity"
  EtherCAT PDO Receive18/1 -> Data Type Conversion10/1  "Actual Position"
  Data Type Conversion10/1 -> Mux4/5
  EtherCAT PDO Receive27/1 -> Data Type Conversion11/1
  Data Type Conversion11/1 -> Mux4/6
  Mux4/1 -> File Log1/1
  EtherCAT PDO Receive8/1 -> Data Type Conversion8/1
  Gain1/1 -> Data Type Conversion6/1  "Demand Current"
  Data Type Conversion8/1 -> Gain1/1
  Data Type Conversion5/1 -> Gain/1
  EtherCAT PDO Receive7/1 -> Data Type Conversion5/1
  Gain/1 -> Data Type Conversion2/1  "Actual Current"
  SV_Target/1 -> Data Type Conversion16/1
  Uc/1 -> Data Type Conversion12/1
  Data Type Conversion12/1 -> Mux3/7
  Data Type Conversion16/1 -> Mux3/6
  EtherCAT PDO Receive28/1 -> Data Type Conversion17/1
  Data Type Conversion17/1 -> [sync]  "sync"
  Stateword/1 -> Data Type Conversion1/1
  [sync] -> Data Type Conversion18/1
  Data Type Conversion18/1 -> Mux3/13

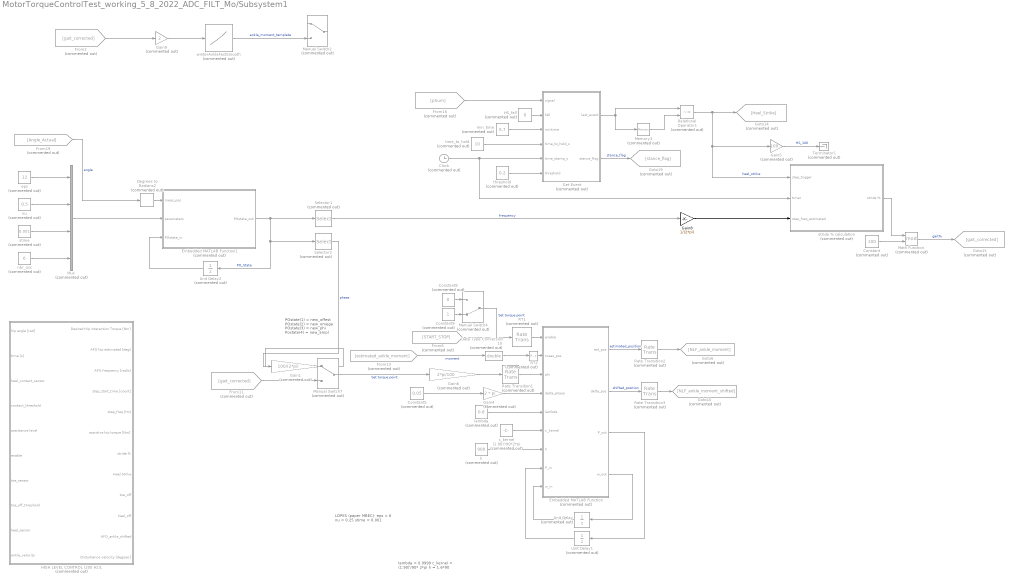
== system MotorTorqueControlTest_working_5_8_2022_ADC_FILT_Mo/Subsystem1 ==
  note: lambda = 0.9999
      | c_kernel = (1:90)'/90* 2*pi
      | h = 1.6*90
  note: LOPES (paper MBEC):
      | eps = 6
      | nu = 0.25
      | stime = 0.001
  note: POstate(1) = new_offest
      | POstate(2) = new_omega
      | POstate(3) = new_phi
      | Postate(4) = new_ampl
  Clock : Clock  Commented=on
  Constant : Constant  Commented=on  Value=100
  Constant5 : Constant  Commented=on  Value=0.05
  Constant8 : Constant  Commented=on  Value=0
  Constant9 : Constant  Commented=on
  Data Type Conversion10 : DataTypeConversion  Commented=on  OutDataTypeStr=double  SaturateOnIntegerOverflow=off  RndMeth=Floor
  Degrees to Radians2 : simulink_extras/Transformations/Degrees to Radians  Commented=on
  Embedded MATLAB Function : MATLAB Function  Commented=on  TreatAsAtomicUnit=on  SystemSampleTime=0.003
  Embedded MATLAB Function1 : MATLAB Function  Commented=on  TreatAsAtomicUnit=on  SystemSampleTime=0.001
  From11 : From  Commented=on  GotoTag=gait_corrected
  From13 : From  Commented=on  GotoTag=estimated_ankle_moment
  From16 : From  Commented=on  GotoTag=pSum
  From19 : From  Commented=on  GotoTag=Angle_Actual
  From2 : From  Commented=on  GotoTag=gait_corrected
  From6 : From  Commented=on  GotoTag=START_STOP
  Gain1 : Gain  Commented=on  Gain=100/(2*pi)
  Gain4 : Gain  Commented=on  Gain=2 * pi
  Gain5 : Gain  Commented=on  Gain=100
  Gain6 : Gain  Commented=on  Gain=2*pi/100
  Gain8 : Gain  Gain=1/(2*pi)
  Gain9 : Gain  Commented=on  Gain=2
  Get Event : Subsystem  Commented=on  TreatAsAtomicUnit=on  SystemSampleTime=1/1000
  Goto10 : Goto  Commented=on  GotoTag=NLF_ankle_moment_shifted
  Goto14 : Goto  Commented=on  GotoTag=Heel_Strike
  Goto15 : Goto  Commented=on  GotoTag=gait_corrected
  Goto19 : Goto  Commented=on  GotoTag=stance_flag
  Goto6 : Goto  Commented=on  GotoTag=NLF_ankle_moment
  HIGH LEVEL CONTROL (200 Hz)1 : Subsystem  Commented=on
  HS_fall : Constant  Commented=on  Value=0
  Manual Switch2 : ManualSwitch  Commented=on
  Manual Switch4 : ManualSwitch  Commented=on  CurrentSetting=0
  Manual Switch7 : ManualSwitch  Commented=on
  Math Function : Math  Commented=on  Operator=mod
  Memory3 : Memory  Commented=on
  Mux : Mux  Commented=on
  RT1 : RateTransition  Commented=on  Deterministic=off  OutPortSampleTime=0.003
  RT2 : RateTransition  Commented=on  Deterministic=off  OutPortSampleTime=0.003
  Rate Transition1 : RateTransition  Commented=on  OutPortSampleTime=0.003
  Rate Transition2 : RateTransition  Commented=on  OutPortSampleTime=0.001
  Rate Transition3 : RateTransition  Commented=on  OutPortSampleTime=0.001
  Relational Operator1 : RelationalOperator  Commented=on  Operator=~=  OutDataTypeStr=boolean  RndMeth=Simplest  InputSameDT=off
  Selector1 : Selector  Commented=on  NumberOfDimensions=2  InputPortWidth=3  IndexOptions=Index vector (dialog),Index vector (dialog)  Indices=2,1  OutputSizes=1,1
  Selector2 : Selector  Commented=on  NumberOfDimensions=2  InputPortWidth=3  IndexOptions=Index vector (dialog),Index vector (dialog)  Indices=3,1  OutputSizes=1,1
  Terminator1 : Terminator  Commented=on
  Unit Delay : UnitDelay  Commented=on  InitialCondition=zeros(90,1)  SampleTime=-1
  Unit Delay1 : UnitDelay  Commented=on  InitialCondition=ones(90,1)  SampleTime=-1
  Unit Delay2 : UnitDelay  Commented=on  InitialCondition=[0;3*pi/2;ones(6,1)*pi/2;zeros(6,1)]  SampleTime=-1
  c_kernel : Constant  Commented=on  Value=(1:90)'/90*2*pi
  eps : Constant  Commented=on  Value=12
  h : Constant  Commented=on  Value=900
  lambda : Constant  Commented=on  Value=0.8
  min_time : Constant  Commented=on  Value=0.7
  nbr_osc : Constant  Commented=on  Value=6
  nu : Constant  Commented=on  Value=0.5
  stime : Constant  Commented=on  Value=0.001
  stride % calculation : Subsystem  Commented=on
  threshold : Constant  Commented=on  Value=0.2
  time_to_hold : Constant  Commented=on  Value=10
  winterAnkleFastSmooth : Lookup  Commented=on  InputValues=[0:200]  Table="[0\t0\t0\t0\t0\t0\t0\t0\t0\t0\t0\t0\t0\t0\t0\t0\t0\t0\t0.0123629052736435\t0.0412585090601981\t0.0720000000000000\t0.104333911147289\t0.137883548612989\t0.172241411772194\t0.207000000000000\t0.241722256560577\t0.275852900274400\t0.308807093851024\t0.340000000000000\t0.368933312610405\t0.395454850289409\t0.419498962823709\t0.441000000000000\t0.459966367997805\t0.476702698567963\t0.491587679854139\t0.505000000000000\t0.517248090398375\t0.528359355438741\t0.538290942759736\t0.547000000000000\t0.554463145408695\t0.560734879677075\t0.565889174106917\t0.570000000000000\t0.573149327966846\t0.575451125852960\t0.577027360812594\t0.578000000000000\t0.578502042723923\t0.578710616911085\t0.578813882642705\t0.579000000000000\t0.579451876137464\t0.580331406502699\t0.581795233616584\t0.584000000000000\t0.587112327726223\t0.591338757078120\t0.596895807890957\t0.604000000000000\t0.612880062957646\t0.623813565184823\t0.637090284819588\t0.653000000000000\t0.671711170443192\t0.692906982182590\t0.716149302830693\t0.741000000000000\t0.767228380269585\t0.795433506084817\t0.826421878857641\t0.861000000000000\t0.899672183478468\t0.941733993478140\t0.986178806738742\t1.03200000000000\t1.07844226081654\t1.12575552000262\t1.17444101918739\t1.22500000000000\t1.27765252325536\t1.33149392651137\t1.38533836651170\t1.43800000000000\t1.48843202116203\t1.53614377395190\t1.58078363976582\t1.62200000000000\t1.65933814209653\t1.69193097768103\t1.71880832442502\t1.73900000000000\t1.75165291045186\t1.75638231532399\t1.75292056253412\t1.74100000000000\t1.72026896609601\t1.69003976102303\t1.64954067543852\t1.59800000000000\t1.53500560016408\t1.46158364058391\t1.37911986071179\t1.28900000000000\t1.19256800824768\t1.09100067664133\t0.985433006714323\t0.877000000000000\t0.767175491845209\t0.658788652850752\t0.555007487430919\t0.459000000000000\t0.373308149371486\t0.297969711955659\t0.232396418562003\t0.176000000000000\t0.128170035668849\t0.0882074993266129\t0.0553912133210702\t0.0290000000000000\t0.00830858295311821\t-0.00742470926211037\t-0.0189456468462838\t-0.0270000000000000\t-0.0322793674813219\t-0.0352586622781714\t-0.0363586259359352\t-0.0360000000000000\t-0.0345973630278306\t-0.0325406416252041\t-0.0302135994099755\t-0.0280000000000000\t-0.0261905554073556\t-0.0247037712210123\t-0.0233651014241628\t-0.0220000000000000\t-0.0204841653427468\t-0.0188942734907467\t-0.0173572448933732\t-0.0160000000000000\t-0.0149196582216572\t-0.0140941348160010\t-0.0134715440023443\t-0.0130000000000000\t-0.0126340767706245\t-0.0123541872452493\t-0.0121472040972494\t-0.0120000000000000\t-0.0119034096958447\t-0.0118641162030018\t-0.0118927646086579\t-0.0120000000000000\t-0.0121897844459966\t-0.0124393479427436\t-0.0127192374681188\t-0.0130000000000000\t-0.0132593275201690\t-0.0135034920260239\t-0.0137459105188668\t-0.0140000000000000\t-0.0142729054733275\t-0.0145466839531609\t-0.0147971204564139\t-0.0150000000000000\t-0.0151334255865212\t-0.0151847721613325\t-0.0151437326554777\t-0.0150000000000000\t-0.0147402671805879\t-0.0143392274015089\t-0.0137685739216755\t-0.0130000000000000\t-0.0120148806911273\t-0.0108333182326318\t-0.00948509665782044\t-0.00800000000000000\t-0.00640333505490292\t-0.00470249966796380\t-0.00290041444704278\t-0.00100000000000000\t0.000987595910738992\t0.00301831690448703\t0.00503987944599156\t0.00700000000000000\t0.00884357641194696\t0.0105042320500157\t0.0119127716630766\t0.0130000000000000\t0.0137162234414732\t0.0140897548954503\t0.0141684089017022\t0.0140000000000000\t0.0136196548221603\t0.0130117483681832\t0.0121479677301145\t0.0110000000000000\t0.00953953226988547\t0.00773825163181676\t0.00556784517783966\t0.00300000000000000]"  SaturateOnIntegerOverflow=off
  wires:
  From2/1 -> Gain9/1
  winterAnkleFastSmooth/1 -> Manual Switch2/2  "ankle_moment_template"
  Gain9/1 -> winterAnkleFastSmooth/1
  Manual Switch7/1 -> Gain6/1  "Set torque point"
  Gain4/1 -> Embedded MATLAB Function/4(delta_phase)
  RT1/1 -> Embedded MATLAB Function/1(enable)
  RT2/1 -> Embedded MATLAB Function/2(meas_pos)
  Embedded MATLAB Function1/1(POstate_out) -> Selector1/1, Unit Delay2/1, Selector2/1  "PO_State"
  Get Event/2(stance_flag) -> Goto19/1  "stance_flag"
  c_kernel/1 -> Embedded MATLAB Function/6(c_kernel)
  From16/1 -> Get Event/1(signal)
  Degrees to Radians2/1 -> Embedded MATLAB Function1/1(meas_pos)
  threshold/1 -> Get Event/6(threshold)
  Mux/1 -> Embedded MATLAB Function1/2(parameters)
  h/1 -> Embedded MATLAB Function/7(h)
  time_to_hold/1 -> Get Event/4(time_to_hold_s)
  nu/1 -> Mux/2
  Selector1/1 -> Gain8/1  "frequency"
  Embedded MATLAB Function/2(delta_pos) -> Rate Transition3/1  "shifted_position"
  Gain5/1 -> Terminator1/1  "HS_100"
  From11/1 -> Manual Switch7/2
  Constant8/1 -> Manual Switch4/1
  Constant5/1 -> Gain4/1
  stride % calculation/1(stride %) -> Math Function/1
  Unit Delay1/1 -> Embedded MATLAB Function/8(P_in)
  Unit Delay/1 -> Embedded MATLAB Function/9(w_in)
  Memory3/1 -> Relational Operator1/2
  From13/1 -> Data Type Conversion10/1  "moment"
  HS_fall/1 -> Get Event/2(fall)
  Selector2/1 -> Gain1/1  "phase"
  Unit Delay2/1 -> Embedded MATLAB Function1/3(POstate_in)
  Rate Transition3/1 -> Goto10/1
  Gain8/1 -> stride % calculation/3(step_freq_estimated)
  Relational Operator1/1 -> Goto14/1, Gain5/1, stride % calculation/1(step_trigger)  "heel_strike"
  Manual Switch4/1 -> RT1/1  "Set torque point"
  lambda/1 -> Embedded MATLAB Function/5(lambda)
  Data Type Conversion10/1 -> RT2/1
  Get Event/1(last_event) -> Relational Operator1/1, Memory3/1
  From19/1 -> Degrees to Radians2/1  "angle"
  min_time/1 -> Get Event/3(mintime)
  stime/1 -> Mux/3
  nbr_osc/1 -> Mux/4
  Rate Transition1/1 -> Embedded MATLAB Function/3(phi)
  Embedded MATLAB Function/4(w_out) -> Unit Delay/1
  Clock/1 -> stride % calculation/2(timer), Get Event/5(time_stamp_s)
  eps/1 -> Mux/1
  Embedded MATLAB Function/1(est_pos) -> Rate Transition2/1  "estimated_position"
  Gain6/1 -> Rate Transition1/1
  Math Function/1 -> Goto15/1  "gait%"
  Rate Transition2/1 -> Goto6/1
  Constant9/1 -> Manual Switch4/2
  Constant/1 -> Math Function/2
  Embedded MATLAB Function/3(P_out) -> Unit Delay1/1
  Gain1/1 -> Manual Switch7/1
  From6/1 -> ?
